simulink model "LATC_Test_Calc3"  (R2021b)
settings: Solver=FixedStepDiscrete  StartTime=0.0  StopTime=inf  FixedStep=0.1  RelTol=1e-3
settings Model: DataDictionary=PubParsGlobal.sldd  Creator=GW00216231  LastModifiedBy=GW00216231
settings SolverCC: AlgebraicLoopSolver=TrustRegion
settings OptimizationCC: DefaultParameterBehavior=Inlined  EnhancedBackFolding=on  PassReuseOutputArgsThreshold=0  OptimizeBlockOrder=speed  DifferentSizesBufferReuse=on  OptimizationCustomize=off
settings DebuggingCC: SignalResolutionControl=TryResolveAllWithWarning  ParameterTunabilityLossMsg=error  SFMachineParentedDataDiag=warning  UnderSpecifiedDimensionMsg=warning
settings SFSimCC: MATLABDynamicMemAlloc=off
settings RTWCC: Description=Vector CANape/vSignalyzer Target (Visual C/C++ Project Makefile)  SystemTargetFile=cnp.tlc  TemplateMakefile=cnp_msdll.tmf
settings CodeAppCC: ForceParamTrailComments=on  OperatorAnnotations=on
settings STFCustomTargetCC: TargetLangStandard=C99 (ISO)  MATLABClassNameForMDSCustomization=Simulink.SoftwareTarget.TargetSpecificTriggerConfigurationBase  SystemTargetFile=cnp.tlc

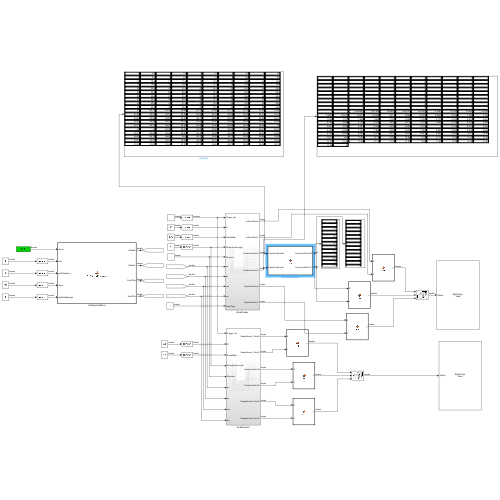
[thumbnail: Simulink's stored preview of the top-level diagram]
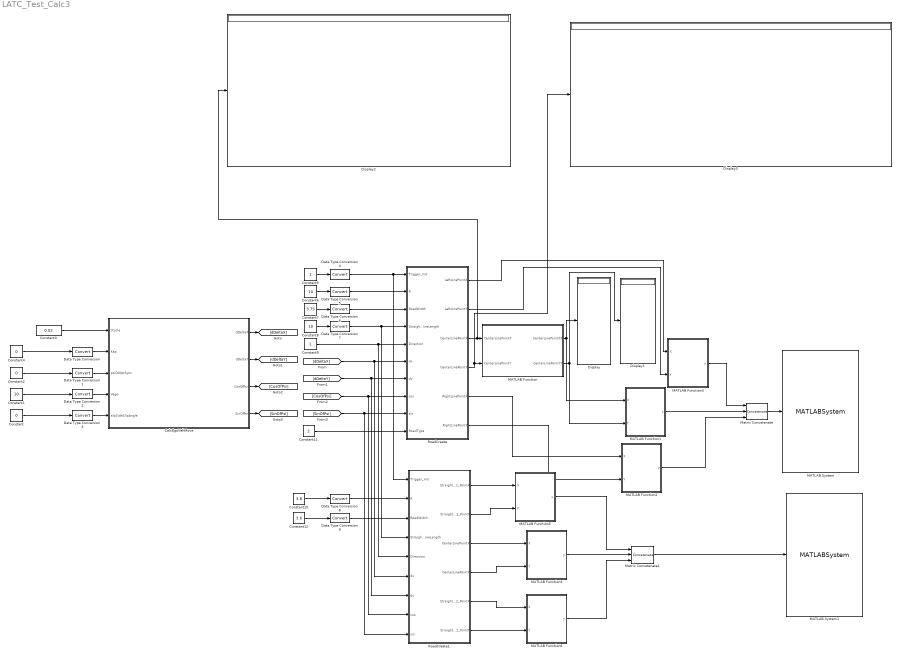
== system LATC_Test_Calc3 ==
  CalcEgoVehMove : MATLAB Function  TreatAsAtomicUnit=on
  Constant : Constant  Value=0
  Constant1 : Constant  Value=10
  Constant10 : Constant  Value=3.8
  Constant11 : Constant  Value=2
  Constant12 : Constant  Value=3.6
  Constant2 : Constant  Value=0
  Constant3 : Constant  Value=0.02
  Constant4 : Constant  Value=0
  Constant5 : Constant
  Constant6 : Constant  Value=10
  Constant7 : Constant  Value=3.75
  Constant8 : Constant  Value=10
  Constant9 : Constant
  Data Type Conversion{,1..9} (10 alike) : DataTypeConversion
  Display{,1..3} (4 alike) : Display
  MATLAB Function : MATLAB Function  TreatAsAtomicUnit=on
  MATLAB Function1 : MATLAB Function  TreatAsAtomicUnit=on
  MATLAB Function2 : MATLAB Function  TreatAsAtomicUnit=on
  MATLAB Function3 : MATLAB Function  TreatAsAtomicUnit=on
  MATLAB Function4 : MATLAB Function  TreatAsAtomicUnit=on
  MATLAB Function5 : MATLAB Function  TreatAsAtomicUnit=on
  MATLAB Function6 : MATLAB Function  TreatAsAtomicUnit=on
  MATLAB System : MATLABSystem  System=BirdsEyeView17a  XLim=[ 0, 120 ]  YLim=[ -30, 30 ]  HasActors=off  ActorsColor=off  HasVision=on  HasRadar=off  HasRoads=off  HasLaneMarkings=off  Camera_Fov=52  Camera_Range=100  Camera_Yaw=0  Camera_Pos=[ 0, 0 ]  Radar_Fov=52  Radar_Range=100  Radar_Yaw=0  Radar_Pos=[ 0, 0 ]  MarkerSize=4  LabelFontSize=4  LabelOffset=[ 1.5, 1.5 ]  aspectratio=off
      mask Type: BirdsEyeView17a
      mask Display:
      | disp(['Bird''s-Eye' char(10) 'View']);
      | port_label('input',1,'Vision');
  MATLAB System1 : MATLABSystem  System=BirdsEyeView17a  XLim=[ 0, 120 ]  YLim=[ -30, 30 ]  HasActors=off  ActorsColor=off  HasVision=on  HasRadar=off  HasRoads=off  HasLaneMarkings=off  Camera_Fov=52  Camera_Range=100  Camera_Yaw=0  Camera_Pos=[ 0, 0 ]  Radar_Fov=52  Radar_Range=100  Radar_Yaw=0  Radar_Pos=[ 0, 0 ]  MarkerSize=4  LabelFontSize=4  LabelOffset=[ 1.5, 1.5 ]  aspectratio=off
      mask Type: BirdsEyeView17a
      mask Display:
      | disp(['Bird''s-Eye' char(10) 'View']);
      | port_label('input',1,'Vision');
  Matrix Concatenate : Concatenate  NumInputs=3  Mode=Multidimensional array
  Matrix Concatenate1 : Concatenate  NumInputs=3  Mode=Multidimensional array
  RoadCreate : Subsystem
  RoadCreate1 : Subsystem
  wires:
  Constant8/1 -> Data Type Conversion7/1
  RoadCreate/3(CenterLinePointX) -> Display2/1, MATLAB Function/1(CenterLinePointX)
  Constant2/1 -> Data Type Conversion1/1
  RoadCreate/4(CenterLinePointY) -> Display3/1, MATLAB Function/2(CenterLinePointY)
  Constant1/1 -> Data Type Conversion2/1
  Data Type Conversion2/1 -> CalcEgoVehMove/4(Vego)
  Data Type Conversion1/1 -> CalcEgoVehMove/3(psiDtOptSync)
  Constant9/1 -> RoadCreate1/5(Direction), RoadCreate/5(Direction)
  CalcEgoVehMove/1(dDeltaX) -> [dDeltaX]
  Constant6/1 -> Data Type Conversion5/1
  [SinOfPsi] -> RoadCreate1/9(sin), RoadCreate/9(sin)
  Constant5/1 -> Data Type Conversion4/1
  Constant7/1 -> Data Type Conversion6/1
  [dDeltaX] -> RoadCreate1/6(dx), RoadCreate/6(dx)
  Constant/1 -> Data Type Conversion3/1
  Constant3/1 -> CalcEgoVehMove/1(tCycle)
  CalcEgoVehMove/4(SinOfPsi) -> [SinOfPsi]
  Data Type Conversion3/1 -> CalcEgoVehMove/5(alpSideSlipAngle)
  [dDeltaY] -> RoadCreate1/7(dy), RoadCreate/7(dy)
  CalcEgoVehMove/3(CosOfPsi) -> [CosOfPsi]
  Data Type Conversion/1 -> CalcEgoVehMove/2(Kap)
  [CosOfPsi] -> RoadCreate1/8(cos), RoadCreate/8(cos)
  CalcEgoVehMove/2(dDeltaY) -> [dDeltaY]
  Data Type Conversion4/1 -> RoadCreate1/1(Trigger_Init), RoadCreate/1(Trigger_Init)
  Data Type Conversion5/1 -> RoadCreate/2(R)
  Data Type Conversion6/1 -> RoadCreate/3(RoadWidth)
  Data Type Conversion7/1 -> RoadCreate1/4(StraightLineLength), RoadCreate/4(StraightLineLength)
  MATLAB Function/1(CenterLinePointXX) -> MATLAB Function1/1(X), Display/1
  RoadCreate/5(RightLinePointX) -> MATLAB Function2/1(X)
  RoadCreate/6(RightLinePointY) -> MATLAB Function2/2(Y)
  RoadCreate/1(LeftLinePointX) -> MATLAB Function3/1(X)
  RoadCreate/2(LeftLinePointY) -> MATLAB Function3/2(Y)
  Matrix Concatenate/1 -> MATLAB System/1
  MATLAB Function3/1(y) -> Matrix Concatenate/1
  MATLAB Function1/1(y) -> Matrix Concatenate/2
  MATLAB Function2/1(y) -> Matrix Concatenate/3
  Constant4/1 -> Data Type Conversion/1
  Constant11/1 -> RoadCreate/10(RoadType)
  RoadCreate1/3(CenterLinePointX) -> MATLAB Function4/1(X)
  RoadCreate1/4(CenterLinePointY) -> MATLAB Function4/2(Y)
  MATLAB Function4/1(y) -> Matrix Concatenate1/2
  Constant10/1 -> Data Type Conversion8/1
  Data Type Conversion8/1 -> RoadCreate1/2(R)
  Constant12/1 -> Data Type Conversion9/1
  Data Type Conversion9/1 -> RoadCreate1/3(RoadWidth)
  RoadCreate1/1(StraightLane1_PointX) -> MATLAB Function5/1(X)
  RoadCreate1/2(StraightLane1_PointY) -> MATLAB Function5/2(Y)
  MATLAB Function5/1(y) -> Matrix Concatenate1/1
  Matrix Concatenate1/1 -> MATLAB System1/1
  RoadCreate1/6(StraightLane2_PointY) -> MATLAB Function6/2(Y)
  RoadCreate1/5(StraightLane2_PointX) -> MATLAB Function6/1(X)
  MATLAB Function6/1(y) -> Matrix Concatenate1/3
  MATLAB Function/2(CenterLinePointYY) -> Display1/1, MATLAB Function1/2(Y)

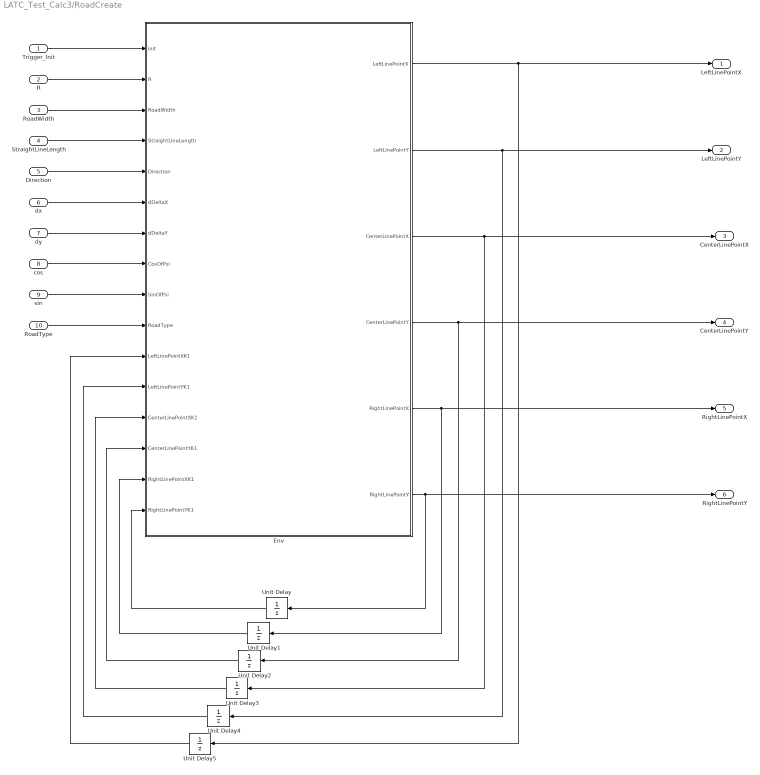
== system LATC_Test_Calc3/RoadCreate ==
  Trigger_Init : Inport
  R : Inport  Port=2
  RoadWidth : Inport  Port=3
  StraightLineLength : Inport  Port=4
  Direction : Inport  Port=5
  dx : Inport  Port=6
  dy : Inport  Port=7
  cos : Inport  Port=8
  sin : Inport  Port=9
  RoadType : Inport  Port=10
  Env : MATLAB Function  TreatAsAtomicUnit=on
  Unit Delay{,1..5} (6 alike) : UnitDelay  SampleTime=-1  HasFrameUpgradeWarning=on
  LeftLinePointX : Outport
  LeftLinePointY : Outport  Port=2
  CenterLinePointX : Outport  Port=3
  CenterLinePointY : Outport  Port=4
  RightLinePointX : Outport  Port=5
  RightLinePointY : Outport  Port=6
  wires:
  Trigger_Init/1 -> Env/1(init)
  R/1 -> Env/2(R)
  RoadWidth/1 -> Env/3(RoadWidth)
  dx/1 -> Env/6(dDeltaX)
  cos/1 -> Env/8(CosOfPsi)
  dy/1 -> Env/7(dDeltaY)
  sin/1 -> Env/9(SinOfPsi)
  Env/6(RightLinePointY) -> RightLinePointY/1, Unit Delay/1
  Unit Delay/1 -> Env/16(RightLinePointYK1)
  Env/5(RightLinePointX) -> RightLinePointX/1, Unit Delay1/1
  Unit Delay1/1 -> Env/15(RightLinePointXK1)
  Env/4(CenterLinePointY) -> CenterLinePointY/1, Unit Delay2/1
  Unit Delay2/1 -> Env/14(CenterLinePointYK1)
  Env/3(CenterLinePointX) -> CenterLinePointX/1, Unit Delay3/1
  Unit Delay3/1 -> Env/13(CenterLinePointXK1)
  Env/2(LeftLinePointY) -> LeftLinePointY/1, Unit Delay4/1
  Unit Delay4/1 -> Env/12(LeftLinePointYK1)
  Env/1(LeftLinePointX) -> LeftLinePointX/1, Unit Delay5/1
  Unit Delay5/1 -> Env/11(LeftLinePointXK1)
  Direction/1 -> Env/5(Direction)
  StraightLineLength/1 -> Env/4(StraightLineLength)
  RoadType/1 -> Env/10(RoadType)

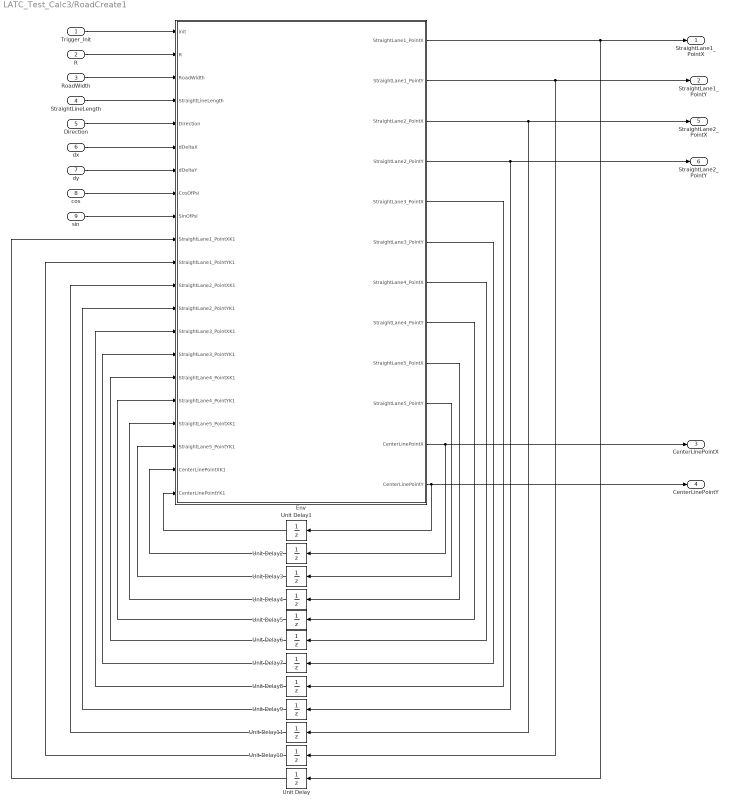
== system LATC_Test_Calc3/RoadCreate1 ==
  Trigger_Init : Inport
  R : Inport  Port=2
  RoadWidth : Inport  Port=3
  StraightLineLength : Inport  Port=4
  Direction : Inport  Port=5
  dx : Inport  Port=6
  dy : Inport  Port=7
  cos : Inport  Port=8
  sin : Inport  Port=9
  Env : MATLAB Function  TreatAsAtomicUnit=on
  Unit Delay{,1..11} (12 alike) : UnitDelay  SampleTime=-1  HasFrameUpgradeWarning=on
  StraightLane1_PointX : Outport
  StraightLane1_PointY : Outport  Port=2
  CenterLinePointX : Outport  Port=3
  CenterLinePointY : Outport  Port=4
  StraightLane2_PointX : Outport  Port=5
  StraightLane2_PointY : Outport  Port=6
  wires:
  StraightLineLength/1 -> Env/4(StraightLineLength)
  Direction/1 -> Env/5(Direction)
  sin/1 -> Env/9(SinOfPsi)
  dy/1 -> Env/7(dDeltaY)
  cos/1 -> Env/8(CosOfPsi)
  dx/1 -> Env/6(dDeltaX)
  RoadWidth/1 -> Env/3(RoadWidth)
  R/1 -> Env/2(R)
  Trigger_Init/1 -> Env/1(init)
  Env/1(StraightLane1_PointX) -> StraightLane1_PointX/1, Unit Delay/1
  Unit Delay/1 -> Env/10(StraightLane1_PointXK1)
  Env/2(StraightLane1_PointY) -> StraightLane1_PointY/1, Unit Delay10/1
  Env/12(CenterLinePointY) -> CenterLinePointY/1, Unit Delay1/1
  Unit Delay1/1 -> Env/21(CenterLinePointYK1)
  Env/11(CenterLinePointX) -> Unit Delay2/1, CenterLinePointX/1
  Unit Delay2/1 -> Env/20(CenterLinePointXK1)
  Env/10(StraightLane5_PointY) -> Unit Delay3/1
  Unit Delay3/1 -> Env/19(StraightLane5_PointYK1)
  Env/9(StraightLane5_PointX) -> Unit Delay4/1
  Unit Delay4/1 -> Env/18(StraightLane5_PointXK1)
  Env/8(StraightLane4_PointY) -> Unit Delay5/1
  Unit Delay5/1 -> Env/17(StraightLane4_PointYK1)
  Env/7(StraightLane4_PointX) -> Unit Delay6/1
  Unit Delay6/1 -> Env/16(StraightLane4_PointXK1)
  Env/6(StraightLane3_PointY) -> Unit Delay7/1
  Unit Delay7/1 -> Env/15(StraightLane3_PointYK1)
  Env/5(StraightLane3_PointX) -> Unit Delay8/1
  Unit Delay8/1 -> Env/14(StraightLane3_PointXK1)
  Env/4(StraightLane2_PointY) -> StraightLane2_PointY/1, Unit Delay9/1
  Unit Delay9/1 -> Env/13(StraightLane2_PointYK1)
  Unit Delay10/1 -> Env/11(StraightLane1_PointYK1)
  Env/3(StraightLane2_PointX) -> StraightLane2_PointX/1, Unit Delay11/1
  Unit Delay11/1 -> Env/12(StraightLane2_PointXK1)

== matlab function LATC_Test_Calc3/RoadCreate1/Env ==
  data: init input boolean; R input; RoadWidth input; StraightLineLength input; Direction input; dDeltaX input; dDeltaY input; CosOfPsi input; SinOfPsi input; StraightLane1_PointX output; StraightLane1_PointXK1 input single; StraightLane1_PointYK1 input single; StraightLane2_PointXK1 input single; StraightLane2_PointYK1 input single; StraightLane3_PointXK1 input single; StraightLane3_PointYK1 input single; StraightLane4_PointXK1 input single; StraightLane4_PointYK1 input single; StraightLane5_PointXK1 input single; StraightLane5_PointYK1 input single; CenterLinePointXK1 input single; CenterLinePointYK1 input single; StraightLane1_PointY output; StraightLane2_PointX output; StraightLane2_PointY output; StraightLane3_PointX output; StraightLane3_PointY output; StraightLane4_PointX output; StraightLane4_PointY output; StraightLane5_PointX output; StraightLane5_PointY output; CenterLinePointX output; CenterLinePointY output
function [StraightLane1_PointX,StraightLane1_PointY,StraightLane2_PointX,StraightLane2_PointY,...
    StraightLane3_PointX,StraightLane3_PointY,StraightLane4_PointX,StraightLane4_PointY,...
    StraightLane5_PointX,StraightLane5_PointY,CenterLinePointX,CenterLinePointY] = ...
    Env(init,R,RoadWidth,StraightLineLength,Direction,dDeltaX,dDeltaY,CosOfPsi,SinOfPsi,...
    StraightLane1_PointXK1,StraightLane1_PointYK1,StraightLane2_PointXK1,StraightLane2_PointYK1,...
    StraightLane3_PointXK1,StraightLane3_PointYK1,StraightLane4_PointXK1,StraightLane4_PointYK1,...
    StraightLane5_PointXK1,StraightLane5_PointYK1,CenterLinePointXK1,CenterLinePointYK1)

CenterLinePointX = single(zeros(300,1));
CenterLinePointY = single(zeros(300,1));

StraightLane1_PointY = single(zeros(100,1));
StraightLane1_PointX = single(zeros(100,1));
StraightLane2_PointY = single(zeros(100,1));
StraightLane2_PointX = single(zeros(100,1));
StraightLane3_PointY = single(zeros(100,1));
StraightLane3_PointX = single(zeros(100,1));
StraightLane4_PointY = single(zeros(100,1));
StraightLane4_PointX = single(zeros(100,1));
StraightLane5_PointY = single(zeros(100,1));
StraightLane5_PointX = single(zeros(100,1));
StraightLane6_PointY = single(zeros(10,1));
StraightLane6_PointX = single(zeros(10,1));

StraightLaneCenter1_PointY = single(zeros(100,1));
StraightLaneCenter1_PointX = single(zeros(100,1));
StraightLaneCenter2_PointY = single(zeros(100,1));
StraightLaneCenter2_PointX = single(zeros(100,1));
CircleLaneCenterPointY = single(zeros(100,1));
CircleLaneCenterPointX = single(zeros(100,1));

StraightLane = StraightLineLength;
boundary_Width = 0.4;
if init==1
    if Direction == 1
        for i = 1:99
            StraightLane1_PointX(i+1) = i*((StraightLane)/single(99));
            StraightLane2_PointX(i+1) = i*((StraightLane)/single(99));
            StraightLane3_PointX(i+1) = i*((StraightLane)/single(99));
            StraightLane4_PointX(i+1) = i*((StraightLane)/single(99));
            StraightLane5_PointX(i+1) = i*((StraightLane)/single(99));
            StraightLaneCenter1_PointX(i+1) = i*((StraightLane)/single(99));
            StraightLaneCenter2_PointX(i+1) = i*((StraightLane)/single(99));
        end

        for i = 1:100
            StraightLane1_PointY(i) = -(RoadWidth/single(2));
            StraightLane2_PointY(i) = (RoadWidth/single(2));
            StraightLane3_PointY(i) = ((RoadWidth/single(2))+boundary_Width);
            StraightLane4_PointY(i) = ((1.5*RoadWidth)+boundary_Width);
            StraightLane5_PointY(i) = ((2.5*RoadWidth)+boundary_Width);
            StraightLaneCenter1_PointY(i) = single(0);
            StraightLaneCenter2_PointY(i) = ((2*RoadWidth)+boundary_Width);
        end

        for i = 1:10
            StraightLane6_PointX(i) = single(StraightLane);
            StraightLane6_PointY(i) = (RoadWidth/single(2))+(i-1)*(boundary_Width/single(9));
        end

        % 画半圆
        for i = 1:100
            CircleLaneCenterPointX(i)=StraightLane+(R)*sin((i-1)*pi/100);
            CircleLaneCenterPointY(i)=R-(R)*cos((i-1)*pi/100);
        end

        CenterLinePointX = [StraightLaneCenter1_PointX;CircleLaneCenterPointX;StraightLaneCenter2_PointX];
        CenterLinePointY = [StraightLaneCenter1_PointY;CircleLaneCenterPointY;StraightLaneCenter2_PointY];

    else
        for i = 1:99
            StraightLane1_PointX(i+1) = i*((StraightLane)/single(99));
            StraightLane2_PointX(i+1) = i*((StraightLane)/single(99));
            StraightLane3_PointX(i+1) = i*((StraightLane)/single(99));
            StraightLane4_PointX(i+1) = i*((StraightLane)/single(99));
            StraightLane5_PointX(i+1) = i*((StraightLane)/single(99));
            StraightLaneCenter1_PointX(i+1) = i*((StraightLane)/single(99));
            StraightLaneCenter2_PointX(i+1) = i*((StraightLane)/single(99));
        end

        for i = 1:100
            StraightLane1_PointY(i) = (RoadWidth/single(2));
            StraightLane2_PointY(i) = -(RoadWidth/single(2));
            StraightLane3_PointY(i) = -((RoadWidth/single(2))+boundary_Width);
            StraightLane4_PointY(i) = -((1.5*RoadWidth)+boundary_Width);
            StraightLane5_PointY(i) = -((2.5*RoadWidth)+boundary_Width);
            StraightLaneCenter1_PointY(i) = single(0);
            StraightLaneCenter2_PointY(i) = -((2*RoadWidth)+boundary_Width);
        end

        for i = 1:10
            StraightLane6_PointX(i) = single(StraightLane);
            StraightLane6_PointY(i) = -(RoadWidth/single(2))-(i-1)*(boundary_Width/single(9));
        end

        for i = 1:100
            CircleLaneCenterPointX(i)=StraightLane+(R)*sin((i-1)*pi/100);
            CircleLaneCenterPointY(i)=-R-(R)*cos((100-i)*pi/100); %注意pi的转向从左到右
        end

        CenterLinePointX = [StraightLaneCenter1_PointX;CircleLaneCenterPointX;StraightLaneCenter2_PointX];
        CenterLinePointY = [StraightLaneCenter1_PointY;CircleLaneCenterPointY;StraightLaneCenter2_PointY];

    end
else
    for i=1:300
        ttt_dx = CenterLinePointXK1(i)-dDeltaX;
        ttt_dy = CenterLinePointYK1(i)-dDeltaY;
        ttt_dxTmp = ttt_dx*CosOfPsi+ttt_dy*SinOfPsi;
        ttt_dyTmp = -ttt_dx*SinOfPsi+ttt_dy*CosOfPsi;
        CenterLinePointX(i) = ttt_dxTmp;
        CenterLinePointY(i) = ttt_dyTmp;
    end
    for i=1:100
        t1_dx = StraightLane1_PointXK1(i)-dDeltaX;
        t1_dy = StraightLane1_PointYK1(i)-dDeltaY;
        t1_dxTmp = t1_dx*CosOfPsi+t1_dy*SinOfPsi;
        t1_dyTmp = -t1_dx*SinOfPsi+t1_dy*CosOfPsi;
        StraightLane1_PointX(i) = t1_dxTmp;
        StraightLane1_PointY(i) = t1_dyTmp;
        t2_dx = StraightLane2_PointXK1(i)-dDeltaX;
        t2_dy = StraightLane2_PointYK1(i)-dDeltaY;
        t2_dxTmp = t2_dx*CosOfPsi+t2_dy*SinOfPsi;
        t2_dyTmp = -t2_dx*SinOfPsi+t2_dy*CosOfPsi;
        StraightLane2_PointX(i) = t2_dxTmp;
        StraightLane2_PointY(i) = t2_dyTmp;
        t3_dx = StraightLane3_PointXK1(i)-dDeltaX;
        t3_dy = StraightLane3_PointYK1(i)-dDeltaY;
        t3_dxTmp = t3_dx*CosOfPsi+t3_dy*SinOfPsi;
        t3_dyTmp = -t3_dx*SinOfPsi+t3_dy*CosOfPsi;
        StraightLane3_PointX(i) = t3_dxTmp;
        StraightLane3_PointY(i) = t3_dyTmp;
        t4_dx = StraightLane4_PointXK1(i)-dDeltaX;
        t4_dy = StraightLane4_PointYK1(i)-dDeltaY;
        t4_dxTmp = t4_dx*CosOfPsi+t4_dy*SinOfPsi;
        t4_dyTmp = -t4_dx*SinOfPsi+t4_dy*CosOfPsi;
        StraightLane4_PointX(i) = t4_dxTmp;
        StraightLane4_PointY(i) = t4_dyTmp;
        t5_dx = StraightLane5_PointXK1(i)-dDeltaX;
        t5_dy = StraightLane5_PointYK1(i)-dDeltaY;
        t5_dxTmp = t5_dx*CosOfPsi+t5_dy*SinOfPsi;
        t5_dyTmp = -t5_dx*SinOfPsi+t5_dy*CosOfPsi;
        StraightLane5_PointX(i) = t5_dxTmp;
        StraightLane5_PointY(i) = t5_dyTmp;
    end
end
%******************************************************************
% Description:  
% param 	 :	
%     	 	   	
% return 	 :	
%******************************************************************

== matlab function LATC_Test_Calc3/MATLAB Function4 ==
  data: X input; y output; Y input
function y = fcn(X,Y)

y = zeros(length(X),9);
for i = 1:1:length(X)
    y(i,1) = X(i);
    y(i,2) = Y(i);
    y(i,3) = 1;
    y(i,4) = 0;
    y(i,5) = 0;
    y(i,6) = i;
    y(i,7) = 0;
    y(i,8) = 1;
end
end

== matlab function LATC_Test_Calc3/MATLAB Function5 ==
  data: X input; y output; Y input
function y = fcn(X,Y)

y = zeros(length(X),9);
for i = 1:1:length(X)
    y(i,1) = X(i);
    y(i,2) = Y(i);
    y(i,3) = 1;
    y(i,4) = 0;
    y(i,5) = 0;
    y(i,6) = i;
    y(i,7) = 0;
    y(i,8) = 1;
end
end

== matlab function LATC_Test_Calc3/MATLAB Function6 ==
  data: X input; y output; Y input
function y = fcn(X,Y)

y = zeros(length(X),9);
for i = 1:1:length(X)
    y(i,1) = X(i);
    y(i,2) = Y(i);
    y(i,3) = 1;
    y(i,4) = 0;
    y(i,5) = 0;
    y(i,6) = i;
    y(i,7) = 0;
    y(i,8) = 1;
end
end

== matlab function LATC_Test_Calc3/CalcEgoVehMove ==
  data: dDeltaX output; tCycle input; Kap input; psiDtOptSync input; Vego input; alpSideSlipAngle input; dDeltaY output; CosOfPsi output; SinOfPsi output
function [dDeltaX,dDeltaY,CosOfPsi,SinOfPsi] = EgoVehicleMovement(tCycle,Kap,psiDtOptSync,Vego,alpSideSlipAngle)
%#codegen
if Kap==0
    dDeltaX = Vego*tCycle;
    dDeltaY = 0;
    CosOfPsi = 1;
    SinOfPsi = 0;
else
    t_kap = Kap;
    if ((Kap>0.125)||(Kap<-0.125))&&(Vego>1)
        t_kapPsiDtSync = psiDtOptSync/Vego;
        if abs(t_kapPsiDtSync)>abs(Kap)
            t_kap = t_kapPsiDtSync;
        end
    end
    t_Psi = t_kap*Vego*tCycle;
    SinOfPsi = sin(t_Psi);
    CosOfPsi = cos(t_Psi);
    t_dDeltaXTemp = SinOfPsi/t_kap;
    t_dDeltaYTemp = 2*(sin(t_Psi/2)*sin(t_Psi/2))/t_kap;
    dDeltaX = cos(alpSideSlipAngle)*t_dDeltaXTemp - sin(alpSideSlipAngle)*t_dDeltaYTemp;
    dDeltaY = sin(alpSideSlipAngle)*t_dDeltaXTemp + cos(alpSideSlipAngle)*t_dDeltaYTemp;
end

== matlab function LATC_Test_Calc3/MATLAB Function2 ==
  data: X input; y output; Y input
function y = fcn(X,Y)

y = zeros(length(X),9);
for i = 1:1:length(X)
    y(i,1) = X(i);
    y(i,2) = Y(i);
    y(i,3) = 1;
    y(i,4) = 0;
    y(i,5) = 0;
    y(i,6) = i;
    y(i,7) = 0;
    y(i,8) = 1;
end
end

== matlab function LATC_Test_Calc3/MATLAB Function ==
  data: CenterLinePointX input; CenterLinePointXX output; CenterLinePointY input; CenterLinePointYY output
function [CenterLinePointXX,CenterLinePointYY]= fcn(CenterLinePointX,CenterLinePointY)
CenterLinePointXX = single(zeros(101,1));
CenterLinePointYY = single(zeros(101,1));
j = 1;
for i = 0:3:300
    if i==0
        i = 1;
    end
    CenterLinePointXX(j,1) = CenterLinePointX(i,1);
    CenterLinePointYY(j,1) = CenterLinePointY(i,1);
    j = j + 1;
end


end

== matlab function LATC_Test_Calc3/MATLAB Function3 ==
  data: X input; y output; Y input
function y = fcn(X,Y)

y = zeros(length(X),9);
for i = 1:1:length(X)
    y(i,1) = X(i);
    y(i,2) = Y(i);
    y(i,3) = 1;
    y(i,4) = 0;
    y(i,5) = 0;
    y(i,6) = i;
    y(i,7) = 0;
    y(i,8) = 1;
end
end

== matlab function LATC_Test_Calc3/RoadCreate/Env ==
  data: init input boolean; R input; RoadWidth input; StraightLineLength input; Direction input; dDeltaX input; dDeltaY input; CosOfPsi input; SinOfPsi input; RoadType input; LeftLinePointX output; LeftLinePointXK1 input single; LeftLinePointYK1 input single; CenterLinePointXK1 input single; CenterLinePointYK1 input single; LeftLinePointY output; RightLinePointXK1 input single; RightLinePointYK1 input single; CenterLinePointX output; CenterLinePointY output; RightLinePointX output; RightLinePointY output
function [LeftLinePointX,LeftLinePointY,CenterLinePointX,CenterLinePointY,RightLinePointX,RightLinePointY] = ...
    Env(init,R,RoadWidth,StraightLineLength,Direction,dDeltaX,dDeltaY,CosOfPsi,SinOfPsi,RoadType,...
    LeftLinePointXK1,LeftLinePointYK1,CenterLinePointXK1,CenterLinePointYK1,RightLinePointXK1,RightLinePointYK1)

% R = single(20);                % m
% RoadWidth = single(3.75);       % m
% StraightLineLength =single(10); %m
% Direction = 1;

% R = R;                % m
% RoadWidth = RoadWidth;       % m
% StraightLineLength =single(10); %m
% Direction = 1;

LeftLinePointX = single(zeros(300,1));
LeftLinePointY = single(zeros(300,1));

CenterLinePointX = single(zeros(300,1));
CenterLinePointY = single(zeros(300,1));

RightLinePointX = single(zeros(300,1));
RightLinePointY = single(zeros(300,1));

LaneLeftPointX = single(zeros(100,1));
LaneLeftPointY = single(zeros(100,1));
LaneRightPointX = single(zeros(100,1));
LaneRightPointY = single(zeros(100,1));
LaneCenterPointX = single(zeros(100,1));
LaneCenterPointY = single(zeros(100,1));

StraightLaneLeft1_PointY = single(zeros(100,1));
StraightLaneLeft1_PointX = single(zeros(100,1));
StraightLaneRight1_PointY = single(zeros(100,1));
StraightLaneRight1_PointX = single(zeros(100,1));
StraightLaneCenter1_PointY = single(zeros(100,1));
StraightLaneCenter1_PointX = single(zeros(100,1));

StraightLaneLeft2_PointY = single(zeros(100,1));
StraightLaneLeft2_PointX = single(zeros(100,1));
StraightLaneRight2_PointY = single(zeros(100,1));
StraightLaneRight2_PointX = single(zeros(100,1));
StraightLaneCenter2_PointY = single(zeros(100,1));
StraightLaneCenter2_PointX = single(zeros(100,1));

StraightLaneLeft3_PointY = single(zeros(100,1));
StraightLaneLeft3_PointX = single(zeros(100,1));
StraightLaneRight3_PointY = single(zeros(100,1));
StraightLaneRight3_PointX = single(zeros(100,1));
CircleLaneCenterPointY = single(zeros(100,1));
CircleLaneCenterPointX = single(zeros(100,1));


if init==1
    switch (RoadType)
        case 1
            if Direction == 1
                for i = 1:100
                    LaneLeftPointX(i)=StraightLineLength+(R+RoadWidth/single(2))*sin((i-1)*pi/100);
                    LaneLeftPointY(i)=R-(R+RoadWidth/single(2))*cos((i-1)*pi/100);
                    LaneRightPointX(i)=StraightLineLength+(R-RoadWidth/single(2))*sin((i-1)*pi/100);
                    LaneRightPointY(i)=R-(R-RoadWidth/single(2))*cos((i-1)*pi/100);

                    LaneCenterPointX(i)=StraightLineLength+(R)*sin((i-1)*pi/100);
                    LaneCenterPointY(i)=R-(R)*cos((i-1)*pi/100);
                end
                for i = 1:99
                    StraightLaneLeft1_PointX(i+1) = i*(StraightLineLength/single(100));
                    StraightLaneRight1_PointX(i+1) = i*(StraightLineLength/single(100));
                    StraightLaneCenter1_PointX(i+1) = i*(StraightLineLength/single(100));

                    StraightLaneLeft2_PointX(i+1) = i*(StraightLineLength/single(100));
                    StraightLaneRight2_PointX(i+1) = i*(StraightLineLength/single(100));
                    StraightLaneCenter2_PointX(i+1) = i*(StraightLineLength/single(100));
                end
                StraightLaneLeft2_PointX = StraightLaneLeft2_PointX(end:-1:1);
                StraightLaneRight2_PointX = StraightLaneRight2_PointX(end:-1:1);
                StraightLaneCenter2_PointX = StraightLaneCenter2_PointX(end:-1:1);
                for i = 1:100
                    StraightLaneLeft1_PointY(i) = -(RoadWidth/single(2));
                    StraightLaneRight1_PointY(i) = (RoadWidth/single(2));
                    StraightLaneLeft2_PointY(i) = single(2)*R+(RoadWidth/single(2));
                    StraightLaneRight2_PointY(i) = single(2)*R-(RoadWidth/single(2));
                    StraightLaneCenter1_PointY(i) = single(0);
                    StraightLaneCenter2_PointY(i) = single(2)*R;

                end

            else
                for i = 1:100
                    LaneLeftPointX(i)=StraightLineLength+(R-RoadWidth/single(2))*sin((100-i)*pi/100);
                    LaneLeftPointY(i)=-R-(R-RoadWidth/single(2))*cos((100-i)*pi/100);

                    LaneRightPointX(i)=StraightLineLength+(R+RoadWidth/single(2))*sin((100-i)*pi/100);
                    LaneRightPointY(i)=-R-(R+RoadWidth/single(2))*cos((100-i)*pi/100);

                    LaneCenterPointX(i)=StraightLineLength+(R)*sin((100-i)*pi/100);
                    LaneCenterPointY(i)=-R-(R)*cos((100-i)*pi/100);
                end
                for i = 1:99
                    StraightLaneLeft1_PointX(i+1) = i*(StraightLineLength/single(100));
                    StraightLaneRight1_PointX(i+1) = i*(StraightLineLength/single(100));
                    StraightLaneCenter1_PointX(i+1) = i*(StraightLineLength/single(100));

                    StraightLaneLeft2_PointX(i+1) = i*(StraightLineLength/single(100));
                    StraightLaneRight2_PointX(i+1) = i*(StraightLineLength/single(100));
                    StraightLaneCenter2_PointX(i+1) = i*(StraightLineLength/single(100));
                end
                StraightLaneLeft2_PointX = StraightLaneLeft2_PointX(end:-1:1);
                StraightLaneRight2_PointX = StraightLaneRight2_PointX(end:-1:1);
                StraightLaneCenter2_PointX = StraightLaneCenter2_PointX(end:-1:1);

                for i = 1:100
                    StraightLaneLeft1_PointY(i) = -(RoadWidth/single(2));
                    StraightLaneRight1_PointY(i) = (RoadWidth/single(2));

                    StraightLaneLeft2_PointY(i) = -single(2)*R+(RoadWidth/single(2));
                    StraightLaneRight2_PointY(i) = -single(2)*R-(RoadWidth/single(2));

                    StraightLaneCenter1_PointY(i) = single(0);
                    StraightLaneCenter2_PointY(i) = -single(2)*R;

                end

            end
            LeftLinePointX = [StraightLaneLeft1_PointX;LaneLeftPointX;StraightLaneLeft2_PointX];
            LeftLinePointY = [StraightLaneLeft1_PointY;LaneLeftPointY;StraightLaneLeft2_PointY];

            CenterLinePointX = [StraightLaneCenter1_PointX;LaneCenterPointX;StraightLaneCenter2_PointX];
            CenterLinePointY = [StraightLaneCenter1_PointY;LaneCenterPointY;StraightLaneCenter2_PointY];

            RightLinePointX = [StraightLaneRight1_PointX;LaneRightPointX;StraightLaneRight2_PointX];
            RightLinePointY = [StraightLaneRight1_PointY;LaneRightPointY;StraightLaneRight2_PointY];
        case 2 
            if Direction == 1
                StraightLine1Length = 50;
                U_Width = 12;
                R = 6;
                RoadWidth = 3.6;
                for i = 1:99
                    StraightLaneLeft1_PointX(i+1) = i*((StraightLine1Length+U_Width)/single(100));
                    StraightLaneRight1_PointX(i+1) = i*((StraightLine1Length)/single(100));
                    StraightLaneCenter1_PointX(i+1) = i*((StraightLine1Length)/single(100));

                    StraightLaneLeft2_PointX(i+1) = i*((StraightLine1Length+U_Width)/single(100));
                    StraightLaneRight2_PointX(i+1) = i*((StraightLine1Length)/single(100));
                    StraightLaneCenter2_PointX(i+1) = i*((StraightLine1Length)/single(100));
                end
                StraightLaneLeft2_PointX = StraightLaneLeft2_PointX(end:-1:1);  %最后的直线倒序
                StraightLaneRight2_PointX = StraightLaneRight2_PointX(end:-1:1);
                StraightLaneCenter2_PointX = StraightLaneCenter2_PointX(end:-1:1);

                for i = 1:100
                    StraightLaneLeft1_PointY(i) = -(RoadWidth/single(2));
                    StraightLaneRight1_PointY(i) = (RoadWidth/single(2));

                    StraightLaneLeft2_PointY(i) = single(2)*R+(RoadWidth/single(2));
                    StraightLaneRight2_PointY(i) = single(2)*R-(RoadWidth/single(2));

                    StraightLaneCenter1_PointY(i) = single(0);
                    StraightLaneCenter2_PointY(i) = single(2)*R;

                    % 两条横线
                    StraightLaneLeft3_PointY(i) = (-(RoadWidth/single(2))) + (i)*((single(2)*R+RoadWidth)/single(100));
                    StraightLaneLeft3_PointX(i) = single((StraightLine1Length+U_Width));

                    StraightLaneRight3_PointY(i) = ((RoadWidth/single(2))) + (i)*((single(2)*R-RoadWidth)/single(100));
                    StraightLaneRight3_PointX(i) = single(StraightLine1Length);
                end
                % 画中心圆弧
                for i = 1:100
                    CircleLaneCenterPointX(i)=StraightLine1Length+(R)*sin((i-1)*pi/100);
                    CircleLaneCenterPointY(i)=R-(R)*cos((i-1)*pi/100);
                end

            else
                StraightLine1Length = 50;
                U_Width = 12;
                R = 6;
                RoadWidth = 3.6;

                for i = 1:99
                    StraightLaneLeft1_PointX(i+1) = i*((StraightLine1Length)/single(100));
                    StraightLaneRight1_PointX(i+1) = i*((StraightLine1Length+U_Width)/single(100));
                    StraightLaneCenter1_PointX(i+1) = i*((StraightLine1Length)/single(100));

                    StraightLaneLeft2_PointX(i+1) = i*((StraightLine1Length)/single(100));
                    StraightLaneRight2_PointX(i+1) = i*((StraightLine1Length+U_Width)/single(100));
                    StraightLaneCenter2_PointX(i+1) = i*((StraightLine1Length)/single(100));
                end
                StraightLaneLeft2_PointX = StraightLaneLeft2_PointX(end:-1:1);  %最后的直线倒序
                StraightLaneRight2_PointX = StraightLaneRight2_PointX(end:-1:1);
                StraightLaneCenter2_PointX = StraightLaneCenter2_PointX(end:-1:1);

                for i = 1:100
                    StraightLaneLeft1_PointY(i) = -(RoadWidth/single(2));
                    StraightLaneRight1_PointY(i) = (RoadWidth/single(2));

                    StraightLaneLeft2_PointY(i) = -single(2)*R+(RoadWidth/single(2));
                    StraightLaneRight2_PointY(i) = -single(2)*R-(RoadWidth/single(2));

                    StraightLaneCenter1_PointY(i) = single(0);
                    StraightLaneCenter2_PointY(i) = -single(2)*R;

                    % 两条横线
                    StraightLaneRight3_PointY(i) = ((RoadWidth/single(2))) - (i)*((single(2)*R+RoadWidth)/single(100));
                    StraightLaneRight3_PointX(i) = single((StraightLine1Length+U_Width));

                    StraightLaneLeft3_PointY(i) = (-(RoadWidth/single(2))) - (i)*((single(2)*R-RoadWidth)/single(100));
                    StraightLaneLeft3_PointX(i) = single(StraightLine1Length);
                end
                % 画中心圆弧
                for i = 1:100
                    CircleLaneCenterPointX(i)=StraightLine1Length+(R)*sin((i-1)*pi/100);
                    CircleLaneCenterPointY(i)=-R-(R)*cos((100-i)*pi/100); %注意pi的转向从左到右
                end

            end
            LeftLinePointX = [StraightLaneLeft1_PointX;StraightLaneLeft3_PointX;StraightLaneLeft2_PointX];
            LeftLinePointY = [StraightLaneLeft1_PointY;StraightLaneLeft3_PointY;StraightLaneLeft2_PointY];

            CenterLinePointX = [StraightLaneCenter1_PointX;CircleLaneCenterPointX;StraightLaneCenter2_PointX];
            CenterLinePointY = [StraightLaneCenter1_PointY;CircleLaneCenterPointY;StraightLaneCenter2_PointY];

            RightLinePointX = [StraightLaneRight1_PointX;StraightLaneRight3_PointX;StraightLaneRight2_PointX];
            RightLinePointY = [StraightLaneRight1_PointY;StraightLaneRight3_PointY;StraightLaneRight2_PointY];

    end


else
    for i=1:300
        t_dx = LeftLinePointXK1(i)-dDeltaX;
        t_dy = LeftLinePointYK1(i)-dDeltaY;
        t_dxTmp = t_dx*CosOfPsi+t_dy*SinOfPsi;
        t_dyTmp = -t_dx*SinOfPsi+t_dy*CosOfPsi;
        LeftLinePointX(i) = t_dxTmp;
        LeftLinePointY(i) = t_dyTmp;

        ttt_dx = CenterLinePointXK1(i)-dDeltaX;
        ttt_dy = CenterLinePointYK1(i)-dDeltaY;
        ttt_dxTmp = ttt_dx*CosOfPsi+ttt_dy*SinOfPsi;
        ttt_dyTmp = -ttt_dx*SinOfPsi+ttt_dy*CosOfPsi;
        CenterLinePointX(i) = ttt_dxTmp;
        CenterLinePointY(i) = ttt_dyTmp;

        tt_dx = RightLinePointXK1(i)-dDeltaX;
        tt_dy = RightLinePointYK1(i)-dDeltaY;
        tt_dxTmp = tt_dx*CosOfPsi+tt_dy*SinOfPsi;
        tt_dyTmp = -tt_dx*SinOfPsi+tt_dy*CosOfPsi;
        RightLinePointX(i) = tt_dxTmp;
        RightLinePointY(i) = tt_dyTmp;
    end
end

== matlab function LATC_Test_Calc3/MATLAB Function1 ==
  data: X input; y output; Y input
function y = fcn(X,Y)

y = zeros(length(X),9);
for i = 1:1:length(X)
    y(i,1) = X(i);
    y(i,2) = Y(i);
    y(i,3) = 1;
    y(i,4) = 0;
    y(i,5) = 0;
    y(i,6) = i;
    y(i,7) = 0;
    y(i,8) = 1;
end
end
